simulink model "current_config"  (R2021b)
settings: Solver=ode4  StartTime=0.0  StopTime=inf  FixedStep=ts  RelTol=1e-3
values from neighbouring files (symbols this model uses):
  ts = 0.0005    [dc_motor_ingps.m]    (also in dc_sim_inpgps.m; in_gps_est.m; untitled.m)
undefined symbols (not defined in the file or in its folder): BlockInfo, ParamInfo, PortInfo, TimeInfo
settings Model: Creator=JongBeom  LastModifiedBy=JongBeom

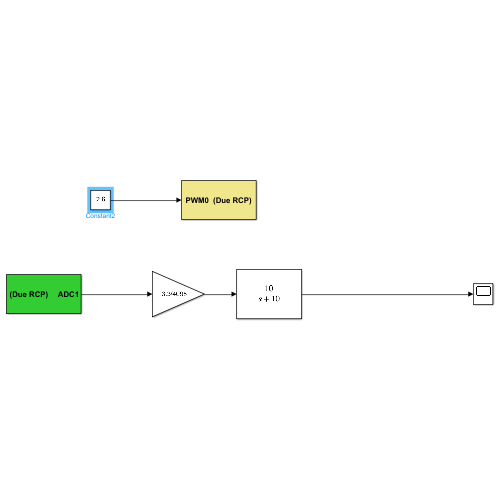
[thumbnail: Simulink's stored preview of the top-level diagram]
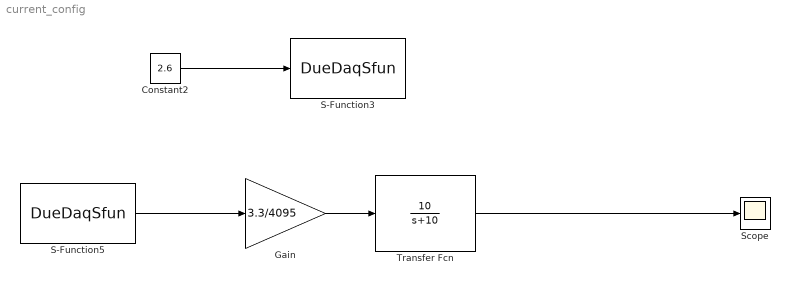
== system current_config ==
  Constant2 : Constant  Value=2.6  SampleTime=ts
  Gain : Gain  Gain=3.3/4095
  S-Function3 : S-Function  FunctionName=DueDaqSfun  Parameters=TimeInfo,BlockInfo,ParamInfo,PortInfo  SFunctionDeploymentMode=off  EnableBusSupport=off  mask(PWM Block){channel=0, method=PWM/Direction, sync=off, freq=20, dead_time=3}
      mask prompts: channel "Channel Number"; sync "Synchronization with Channel 0"; freq "Frequency (KHz)"; dead_time "Dead Time"
      mask help: Send PWM information to Arduino Due
      mask init:
      | DueDaqRcp_PWM_callback;
      mask TypeOptions channel: 0 | 1 | 2 | 3 | 4 | 5
      mask Callback channel: DueDaqRcp_PWM_callback;
      mask TypeOptions method: PWM/Direction | Complementary PWM
      mask Callback method: DueDaqRcp_PWM_callback;
      mask TypeOptions freq: 1 | 10 | 20
      mask Display:
      | color('black');text(0.95,0.5,'(Due RCP)','horizontalalignment','right');
      | color('black');port_label('input', 1,  ' PWM0')
  S-Function5 : S-Function  FunctionName=DueDaqSfun  Parameters=TimeInfo,BlockInfo,ParamInfo,PortInfo  SFunctionDeploymentMode=off  EnableBusSupport=off  mask(ADC Block){channel=1}
      mask prompts: channel "Channel Number"
      mask help: Receive ADC data from Arduino Due
      mask init:
      | DueDaqRcp_ADC_callback;
      mask TypeOptions channel: 0 | 1 | 2 | 3 | 4 | 5 | 6 | 7
      mask Display:
      | color('black');text(0.05,0.5,'(Due RCP)','horizontalalignment','left');
      | color('black');port_label('output', 1,  ' ADC1')
  Scope : Scope
  Transfer Fcn : TransferFcn  Numerator=[10]  Denominator=[1 10]
  wires:
  S-Function5/1 -> Gain/1
  Gain/1 -> Transfer Fcn/1
  Transfer Fcn/1 -> Scope/1
  Constant2/1 -> S-Function3/1
